simulink model "Cart_Pendulum_Linearised_a_n9945008"  (R2018b)
settings: Solver=VariableStepAuto  StartTime=0.0  StopTime=10.0  RelTol=1e-3
values from neighbouring files (symbols this model uses):
  g = 9.81    [MainFile_Linearised_a_n9945008.m]
  l = 0.2    [MainFile_Linearised_a_n9945008.m]
  m = 0.15    [MainFile_Linearised_a_n9945008.m]
  Mc = 0.4    [MainFile_Linearised_a_n9945008.m]
settings Model: Creator=Cody  LastModifiedBy=Cody

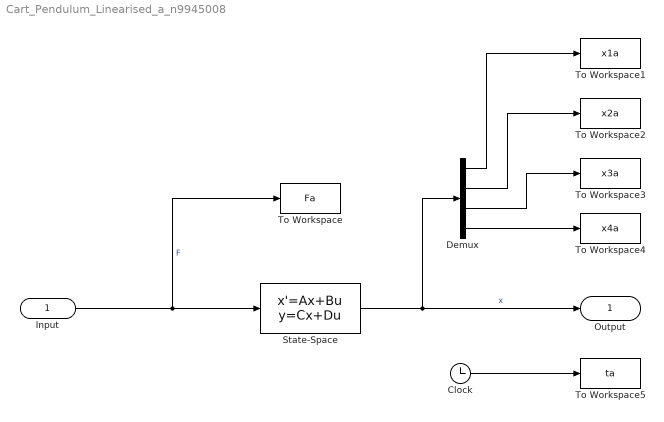
== system Cart_Pendulum_Linearised_a_n9945008 ==
  Input : Inport
  Clock : Clock
  Demux : Demux
  State-Space : StateSpace  A=[0,0,1,0;0,0,0,1;0,-(g*m)/Mc,0,0;0,(g*(Mc+m))/l*Mc,0,0]  B=[0;0;1/Mc;1/l*Mc]  C=eye(4)  D=zeros(4,1)  InitialCondition=[0;pi/180;0;0]
  To Workspace : ToWorkspace  VariableName=Fa  SaveFormat=Timeseries  SampleTime=-1
  To Workspace1 : ToWorkspace  VariableName=x1a  SampleTime=-1
      settings: Save2DSignal=2-D array (concatenate along first dimension)
  To Workspace2 : ToWorkspace  VariableName=x2a  SampleTime=-1
      settings: Save2DSignal=2-D array (concatenate along first dimension)
  To Workspace3 : ToWorkspace  VariableName=x3a  SampleTime=-1
      settings: Save2DSignal=2-D array (concatenate along first dimension)
  To Workspace4 : ToWorkspace  VariableName=x4a  SampleTime=-1
      settings: Save2DSignal=2-D array (concatenate along first dimension)
  To Workspace5 : ToWorkspace  VariableName=ta  SampleTime=-1
      settings: Save2DSignal=2-D array (concatenate along first dimension)
  Output : Outport
  wires:
  Input/1 -> To Workspace/1, State-Space/1  "F"
  State-Space/1 -> Demux/1, Output/1  "x"
  Demux/1 -> To Workspace1/1
  Demux/2 -> To Workspace2/1
  Demux/3 -> To Workspace3/1
  Demux/4 -> To Workspace4/1
  Clock/1 -> To Workspace5/1
